simulink model "Plant_inversion_nominal_single_P"  (R2019b)
settings: Solver=ode3  StartTime=-8.75  StopTime=10.0  FixedStep=0.001  RelTol=1e-3
settings Model: Creator=Aurelio Piazzi  LastModifiedBy=Aurus

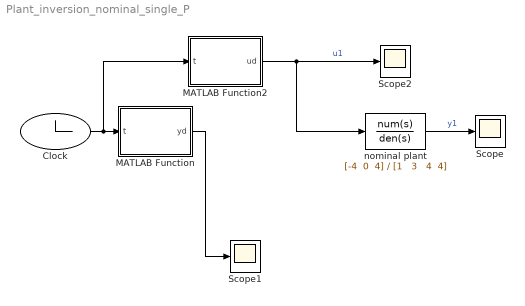
== system Plant_inversion_nominal_single_P ==
  Clock : Clock
  MATLAB Function : MATLAB Function  TreatAsAtomicUnit=on
  MATLAB Function2 : MATLAB Function  TreatAsAtomicUnit=on
  Scope : Scope
  Scope1 : Scope
  Scope2 : Scope
  nominal plant : TransferFcn  Numerator="[-4  0  4]"  Denominator="[1   3   4  4]"
  wires:
  MATLAB Function/1(yd) -> Scope1/1
  nominal plant/1 -> Scope/1  "y1"
  Clock/1 -> MATLAB Function2/1(t), MATLAB Function/1(t)
  MATLAB Function2/1(ud) -> nominal plant/1, Scope2/1  "u1"

== matlab function Plant_inversion_nominal_single_P/MATLAB Function ==
  data: t input; yd output
function yd = yd(t)
 if(t<0)
     yd = 0;
 elseif (t<3)
     yd = (1/3)*t^2-(2/27)*t^3;
 else
     yd = 1;
 end

== matlab function Plant_inversion_nominal_single_P/MATLAB Function2 ==
  data: t input; ud output
function ud = ud(t)
 if(t<0)
     ud = (1/3)*exp(t)+(5/3)*exp(t-3);
 elseif (t<3)
     ud = -(1/9)*t+(1/9)*t^2-(2/27)*t^3-(5/18)*exp(-t)+11/18+(5/3)*exp(t-3);
 else
     ud = 1-(5/18)*exp(-t)-(1/18)*exp(3-t);
 end
